simulink model "Model_2"  (R2017b)
settings: Solver=ode45  StartTime=0.0  StopTime=3000  MaxStep=0.1  RelTol=1e-3
values from neighbouring files (symbols this model uses):
  A = 2    [Model_1_Konstanten.m]
  ROHL = 1.225    [Model_1_Konstanten.m]
undefined symbols (not defined in the file or in its folder): sigbuilder_block
settings Model: Creator=lukasschwoerer  LastModifiedBy=lukasschwoerer

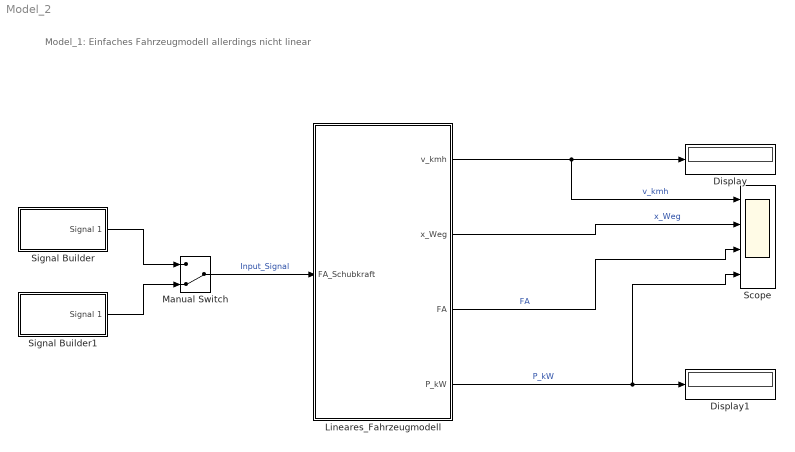
== system Model_2 ==
  note: Model_1: Einfaches Fahrzeugmodell allerdings nicht linear
  Display : Display
  Display1 : Display
  Lineares_Fahrzeugmodell : Subsystem  mask{m=500, cW=0.35}
      mask prompts: m "Fahrzeugmasse"; cW "Luftwiederstandsbeiwert"
  Manual Switch : ManualSwitch  CurrentSetting=0
  Scope : Scope  NumInputPorts=4
  Signal Builder : Subsystem  Tag=STV Subsys  LoadFcn=sigbuilder_block('load');  StartFcn=sigbuilder_block('start');  StopFcn=sigbuilder_block('stop');  ClipboardFcn=sigbuilder_block('clipboard');  mask(Sigbuilder block){tuvar=[0:10]}
      mask help: Simulink:masks:SigbuilderBlock_MD
      mask init:
      | if ~strcmp(get_param(bdroot(gcbh),'SimulationStatus'),'stopped') tuvar = sigbuilder_block('maskInit'); end
      settings: CopyFcn=sigbuilder_block('copy');  DeleteFcn=sigbuilder_block('delete');  ModelCloseFcn=sigbuilder_block('modelClose');  PreSaveFcn=sigbuilder_block('preSave');  PauseFcn=sigbuilder_block('pause');  ContinueFcn=sigbuilder_block('continue');  NameChangeFcn=sigbuilder_block('namechange');  OpenFcn=sigbuilder_block('open',[259 119 1060 556 ]);  CloseFcn=sigbuilder_block('close');
      mask Display: plot(0, 0, 100, 100,[2, 2, 32, 32, 2], [68, 8, 8, 68, 68],[32, 2], [38, 38], [32, 19, 2],[53, 60, 44], [32, 17, 17, 2],[16, 16, 31, 31]);txt = getActiveGroup(gcbh);text(2, 100, txt,'verticalAlignment', 'top');
  Signal Builder1 : Subsystem  Tag=STV Subsys  LoadFcn=sigbuilder_block('load');  StartFcn=sigbuilder_block('start');  StopFcn=sigbuilder_block('stop');  ClipboardFcn=sigbuilder_block('clipboard');  mask(Sigbuilder block){tuvar=[0:10]}
      mask help: Simulink:masks:SigbuilderBlock_MD
      mask init:
      | if ~strcmp(get_param(bdroot(gcbh),'SimulationStatus'),'stopped') tuvar = sigbuilder_block('maskInit'); end
      settings: CopyFcn=sigbuilder_block('copy');  DeleteFcn=sigbuilder_block('delete');  ModelCloseFcn=sigbuilder_block('modelClose');  PreSaveFcn=sigbuilder_block('preSave');  PauseFcn=sigbuilder_block('pause');  ContinueFcn=sigbuilder_block('continue');  NameChangeFcn=sigbuilder_block('namechange');  OpenFcn=sigbuilder_block('open',[31 142 1157 663 ]);  CloseFcn=sigbuilder_block('close');
      mask Display: plot(0, 0, 100, 100,[2, 2, 32, 32, 2], [68, 8, 8, 68, 68],[32, 2], [38, 38], [32, 19, 2],[53, 60, 44], [32, 17, 17, 2],[16, 16, 31, 31]);txt = getActiveGroup(gcbh);text(2, 100, txt,'verticalAlignment', 'top');
  wires:
  Signal Builder/1(Signal 1) -> Manual Switch/1
  Signal Builder1/1(Signal 1) -> Manual Switch/2
  Lineares_Fahrzeugmodell/1(v_kmh) -> Display/1, Scope/1  "v_kmh"
  Manual Switch/1 -> Lineares_Fahrzeugmodell/1(FA_Schubkraft)  "Input_Signal"
  Lineares_Fahrzeugmodell/2(x_Weg) -> Scope/2  "x_Weg"
  Lineares_Fahrzeugmodell/3(FA) -> Scope/3  "FA"
  Lineares_Fahrzeugmodell/4(P_kW) -> Scope/4, Display1/1  "P_kW"

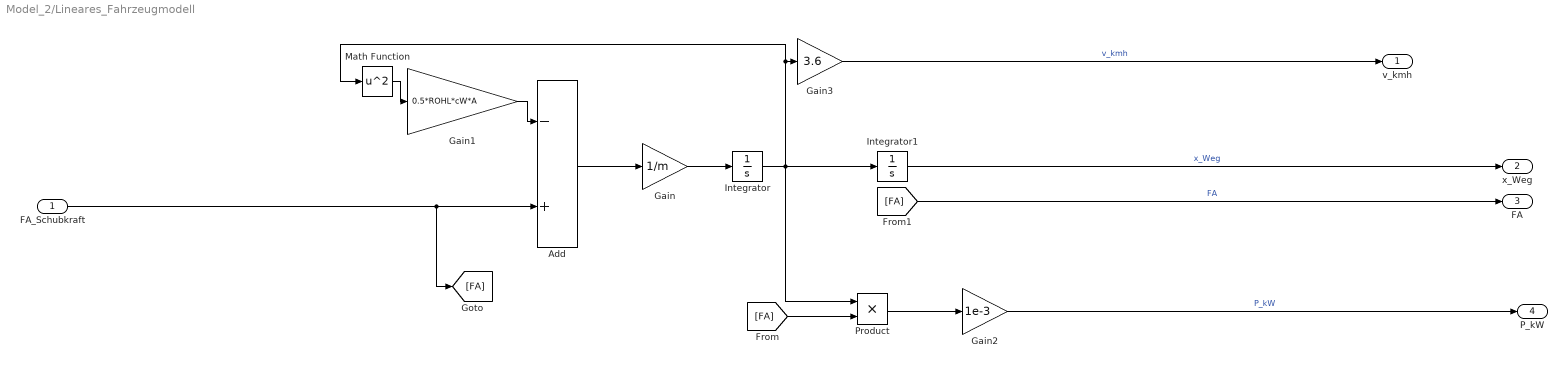
== system Model_2/Lineares_Fahrzeugmodell ==
  FA_Schubkraft : Inport
  Add : Sum  Inputs=-+
  Gain : Gain  Gain=1/m
  Gain1 : Gain  Gain=0.5*ROHL*cW*A
  Gain2 : Gain  Gain=1e-3
  Gain3 : Gain  Gain=3.6
  Integrator : Integrator
  Integrator1 : Integrator
  Math Function : Math  Operator=square  SaturateOnIntegerOverflow=on
  Product : Product
  v_kmh : Outport
  x_Weg : Outport  Port=2
  FA : Outport  Port=3
  P_kW : Outport  Port=4
  wires:
  Gain1/1 -> Add/1
  Gain2/1 -> P_kW/1  "P_kW"
  Gain3/1 -> v_kmh/1  "v_kmh"
  [FA] -> Product/2
  Add/1 -> Gain/1
  Gain/1 -> Integrator/1
  Integrator1/1 -> x_Weg/1  "x_Weg"
  [FA] -> FA/1  "FA"
  Product/1 -> Gain2/1
  FA_Schubkraft/1 -> [FA], Add/2
  Integrator/1 -> Math Function/1, Gain3/1, Integrator1/1, Product/1
  Math Function/1 -> Gain1/1

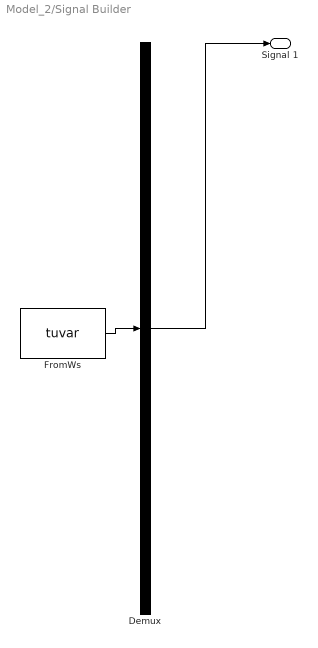
== system Model_2/Signal Builder ==
  Demux : Demux  Tag=STV Demux  Outputs=1
  FromWs : FromWorkspace  Tag=STV FromWs  VariableName=tuvar  SampleTime=0
      SigBuilderData=|
      | common.afterFinalStr = 'Extrapolate'
      | common.sampleTime = 0
      | dataSet.timeRange = [0 100]
      | dataSet.name = 'Group 1'
      | sbobj.Groups.Name = 'Group 1'
      | sbobj.Groups.Signals.Name = 'Signal 1'
      | sbobj.Groups.Signals.XData = [0 10 100]
      | sbobj.Groups.Signals.YData = [0 800 800]
      | sbobj.Groups.TimeRange = [0 100]
  Signal 1 : Outport  Tag=STV Outport
  wires:
  Demux/1 -> Signal 1/1
  FromWs/1 -> Demux/1

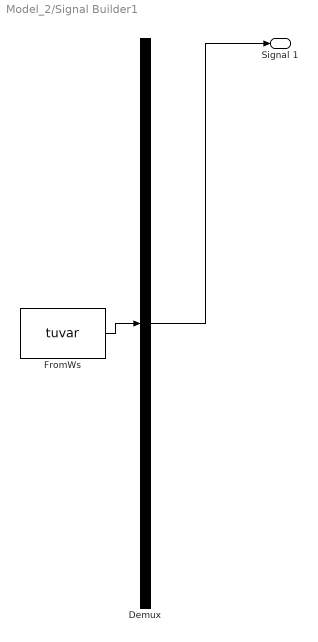
== system Model_2/Signal Builder1 ==
  Demux : Demux  Tag=STV Demux  Outputs=1
  FromWs : FromWorkspace  Tag=STV FromWs  VariableName=tuvar  SampleTime=0
      SigBuilderData=|
      | common.afterFinalStr = 'Extrapolate'
      | common.sampleTime = 0
      | dataSet.timeRange = [0 3000]
      | dataSet.name = 'Group 1'
      | sbobj.Groups.Name = 'Group 1'
      | sbobj.Groups.Signals.Name = 'Signal 1'
      | sbobj.Groups.Signals.XData = [0 10 1000 1010 3000]
      | sbobj.Groups.Signals.YData = [0 800 800 0 0]
      | sbobj.Groups.TimeRange = [0 3000]
  Signal 1 : Outport  Tag=STV Outport
  wires:
  Demux/1 -> Signal 1/1
  FromWs/1 -> Demux/1
